simulink model "HomeWork4_Koundinya"  (Simulink 8.2)
settings: Solver=FixedStepDiscrete  StartTime=0.0  StopTime=10  FixedStep=Ts  RelTol=1e-3
values from neighbouring files (symbols this model uses):
  amp = 0.3    [Main.m]
  den = [1 Thetaupdate(1:na,1)']    [Koundinya_RLSE.m]    (also in Koundinya_ThetaIV4.m = [1 Thetaiv4(1:na,1)']; Main.m = [1 0.8 0.2])
  num = [Thetaupdate(na+1:N1)']    [Koundinya_RLSE.m]    (also in Koundinya_ThetaIV4.m = [Thetaiv4(na+1:N1)']; Main.m = [0.5 0.1])
  Ts = 0.1    [Main.m]
libraries: simulink x2
settings Model: Creator=BDawson2  LastModifiedBy=Pranav
settings OptimizationCC: InitFltsAndDblsToZero=on
settings DebuggingCC: SaveWithParameterizedLinksMsg=none
settings GRTTargetCC: TargetFcnLib=ansi_tfl_tmw.mat

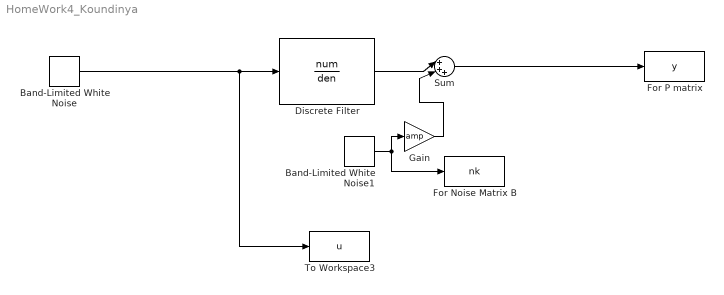
== system HomeWork4_Koundinya ==
  Band-Limited White Noise : simulink/Sources/Band-Limited White Noise  Cov=1  Ts=Ts  seed=[23341]
  Band-Limited White Noise1 : simulink/Sources/Band-Limited White Noise  Cov=amp  Ts=Ts  seed=[30000]
  Discrete Filter : DiscreteFilter  Numerator=num  Denominator=den
  For Noise Matrix B : ToWorkspace  VariableName=nk  SampleTime=-1
  For P matrix : ToWorkspace  VariableName=y  SampleTime=-1
  Gain : Gain  Gain=amp
  Sum : Sum  Inputs=|+++
  To Workspace3 : ToWorkspace  VariableName=u  SampleTime=-1
  wires:
  Band-Limited White Noise/1 -> To Workspace3/1, Discrete Filter/1
  Band-Limited White Noise1/1 -> For Noise Matrix B/1, Gain/1
  Discrete Filter/1 -> Sum/1
  Sum/1 -> For P matrix/1
  Gain/1 -> Sum/2
